simulink model "MatrixToolsEx"  (R2015a)
settings: Solver=ode45  StartTime=0.0  StopTime=10.0  RelTol=1e-3
libraries: lib_GenTools_MinMax x3, lib_GenTools_SubMatrix x1
settings Model: Creator=jlkratz  LastModifiedBy=jlkratz

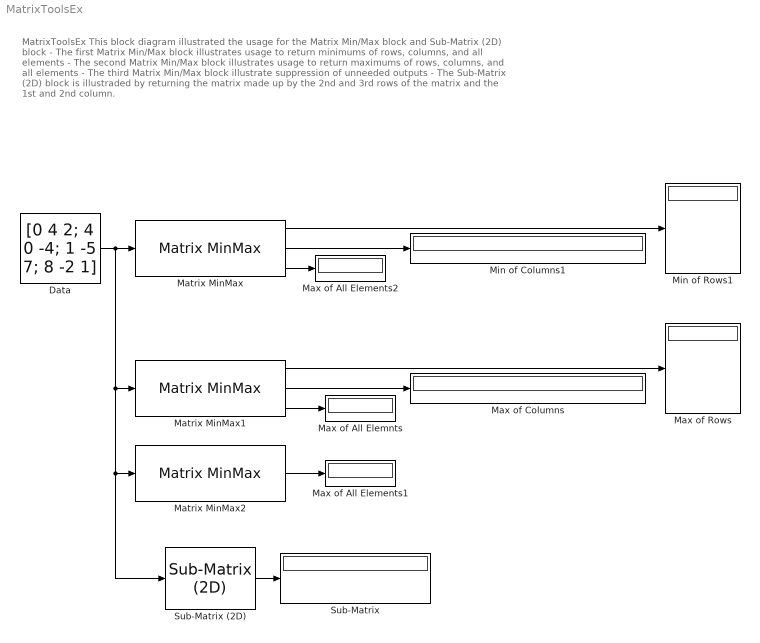
== system MatrixToolsEx ==
  note: MatrixToolsEx
      |
      | This block diagram illustrated the usage for the Matrix Min/Max block and Sub-Matrix (2D) block
      | - The first Matrix Min/Max block illustrates usage to return minimums of rows, columns, and all
      | elements
      | - The second Matrix Min/Max block illustrates usage to return maximums of rows, columns, and all
      | elements
      | - The third Matrix Min/Max block illustrate suppression of unneeded outputs
      | - The Sub-Matrix (2D) block is illustraded by returning the matrix made up by the 2nd and 3rd rows
      | of the matrix and the 1st and 2nd column.
  Data : Constant  Value=[0 4 2; 4 0 -4; 1 -5 7; 8 -2 1]
  Matrix MinMax : lib_GenTools_MinMax/Matrix MinMax  rows_M=on  cols_M=on  all_M=on  minmax_M=on  BN_M=gcb
  Matrix MinMax1 : lib_GenTools_MinMax/Matrix MinMax  rows_M=on  cols_M=on  all_M=on  minmax_M=off  BN_M=gcb
  Matrix MinMax2 : lib_GenTools_MinMax/Matrix MinMax  rows_M=off  cols_M=off  all_M=on  minmax_M=off  BN_M=gcb
  Max of All Elements1 : Display
  Max of All Elements2 : Display
  Max of All Elemnts : Display
  Max of Columns : Display
  Max of Rows : Display
  Min of Columns1 : Display
  Min of Rows1 : Display
  Sub-Matrix : Display
  Sub-Matrix (2D) : lib_GenTools_SubMatrix/Sub-Matrix (2D)  R1_M=2  R2_M=3  C1_M=1  C2_M=2  BN_M=double(gcb)
  wires:
  Sub-Matrix (2D)/1 -> Sub-Matrix/1
  Data/1 -> Matrix MinMax1/1, Matrix MinMax2/1, Sub-Matrix (2D)/1, Matrix MinMax/1
  Matrix MinMax2/1 -> Max of All Elements1/1
  Matrix MinMax1/3 -> Max of All Elemnts/1
  Matrix MinMax1/2 -> Max of Columns/1
  Matrix MinMax1/1 -> Max of Rows/1
  Matrix MinMax/2 -> Min of Columns1/1
  Matrix MinMax/1 -> Min of Rows1/1
  Matrix MinMax/3 -> Max of All Elements2/1
